simulink model "model"  (Simulink 7.3)
settings: Solver=ode45  StartTime=0.0  StopTime=2  RelTol=1e-3
values from neighbouring files (symbols this model uses):
  C_bp = 0.358    [init.m]
  C_bv = 10.71    [init.m]
  C_ep = 0.668    [init.m]
  C_ev = 20    [init.m]
  C_hp = 0.119    [init.m]
  C_hv = 3.57    [init.m]
  C_la = 19.23    [init.m]
  C_mp = 0.525    [init.m]
  C_mv = 15.71    [init.m]
  C_pa = 0.76    [init.m]
  C_pp = 5.8    [init.m]
  C_pv = 25.37    [init.m]
  C_ra = 31.25    [init.m]
  C_sa = 0.28    [init.m]
  C_sp = 2.05    [init.m]
  C_sv = 61.11    [init.m]
  D_E_max_lv = 2    [init.m]
  D_E_max_rv = 2    [init.m]
  D_R_ep = 2    [init.m]
  D_R_mp = 2    [init.m]
  D_R_sp = 2    [init.m]
  D_T_s = 2    [init.m]
  D_T_v = 0.02    [init.m]
  D_u_ev = 5    [init.m]
  D_u_mv = 5    [init.m]
  D_u_sv = 5    [init.m]
  D_v = 6    [init.m]
  E_max_lv_0 = 2.392    [init.m]
  E_max_rv_0 = 1.412    [init.m]
  f_ab_0 = 1    [init.m]
  f_abmax = 47.78    [init.m]
  f_abmin = 0    [init.m]
  f_ac_max = 17.07    [init.m]
  f_ac_min = 0    [init.m]
  f_ac_n = 3.6    [init.m]
  f_es_0 = 16.11    [init.m]
  f_es_inf = 2.1    [init.m]
  f_es_max = 60    [init.m]
  f_es_min = 0    [init.m]
  f_ev_0 = 3.2    [init.m]
  f_ev_inf = 6.3    [init.m]
  fi_sh = 0    [init.m]
  fi_sp = 0    [init.m]
  fi_v = -0.68    [init.m]
  G_ap = 23.29    [init.m]
  G_E_max_lv = 0.475    [init.m]
  G_E_max_rv = 0.282    [init.m]
  G_R_ep = 1.94    [init.m]
  G_R_mp = 2.47    [init.m]
  G_R_sp = 0.695    [init.m]
  G_T_s = -0.13    [init.m]
  G_T_v = 0.09    [init.m]
  G_u_ev = -74.21    [init.m]
  G_u_mv = -58.29    [init.m]
  G_u_sv = -265.4    [init.m]
  G_v = 0.125    [init.m]
  k_a_b = 11.76    [init.m]
  k_ac = 29.27    [init.m]
  k_e_lv = 0.014    [init.m]
  k_e_rv = 0.011    [init.m]
  k_es = 0.0675    [init.m]
  k_ev = 7.06    [init.m]
  k_r_lv = 0.000375    [init.m]
  k_r_rv = 0.0014    [init.m]
  k_sys = 0.075    [init.m]
  L_pa = 0.00018    [init.m]
  p_as_o2 = 30    [init.m]
  p_as_o2_n = 45    [init.m]
  p_n = 92    [init.m]
  P_o_lv = 1.5    [init.m]
  P_o_rv = 1.5    [init.m]
  R_bp = 6.57    [init.m]
  R_bv = 0.075    [init.m]
  R_ep_0 = 1.655    [init.m]
  R_ev = 0.04    [init.m]
  R_hp = 19.71    [init.m]
  R_hv = 0.224    [init.m]
  R_la = 0.0025    [init.m]
  R_mp_0 = 2.106    [init.m]
  R_mv = 0.05    [init.m]
  R_pa = 0.023    [init.m]
  R_pp = 0.0894    [init.m]
  R_pv = 0.0056    [init.m]
  R_ra = 0.0025    [init.m]
  R_sa = 0.06    [init.m]
  R_sp_0 = 2.49    [init.m]
  R_sv = 0.038    [init.m]
  T_0 = 0.58    [init.m]
  T_sys_0 = 0.5    [init.m]
  tau_c = 2    [init.m]
  tau_E_max_rv = 8    [init.m]
  tau_p = 2    [init.m]
  tau_pb = 2.076    [init.m]
  tau_R_ep = 6    [init.m]
  tau_R_mp = 6    [init.m]
  tau_R_sp = 6    [init.m]
  tau_T_s = 2    [init.m]
  tau_T_v = 1.5    [init.m]
  tau_u_ev = 20    [init.m]
  tau_u_mv = 20    [init.m]
  tau_u_sv = 20    [init.m]
  tau_v = 3    [init.m]
  tau_zb = 6.37    [init.m]
  V_tn = 0.583    [init.m]
  V_tot = 5300    [init.m]
  V_u_bp = 72.13    [init.m]
  V_u_bv = 294.64    [init.m]
  V_u_ep = 134.64    [init.m]
  V_u_ev_0 = 640.73    [init.m]
  V_u_hp = 24    [init.m]
  V_u_hv = 98.21    [init.m]
  V_u_la = 25    [init.m]
  V_u_lv = 16.77    [init.m]
  V_u_mp = 105.8    [init.m]
  V_u_mv_0 = 503.26    [init.m]
  V_u_pa = 0    [init.m]
  V_u_pp = 123    [init.m]
  V_u_pv = 120    [init.m]
  V_u_ra = 25    [init.m]
  V_u_rv = 40.8    [init.m]
  ... (+11 more)
(part 1 of 2)
settings Model: Creator=Mirek Muzny  LastModifiedBy=Mirek Muzny

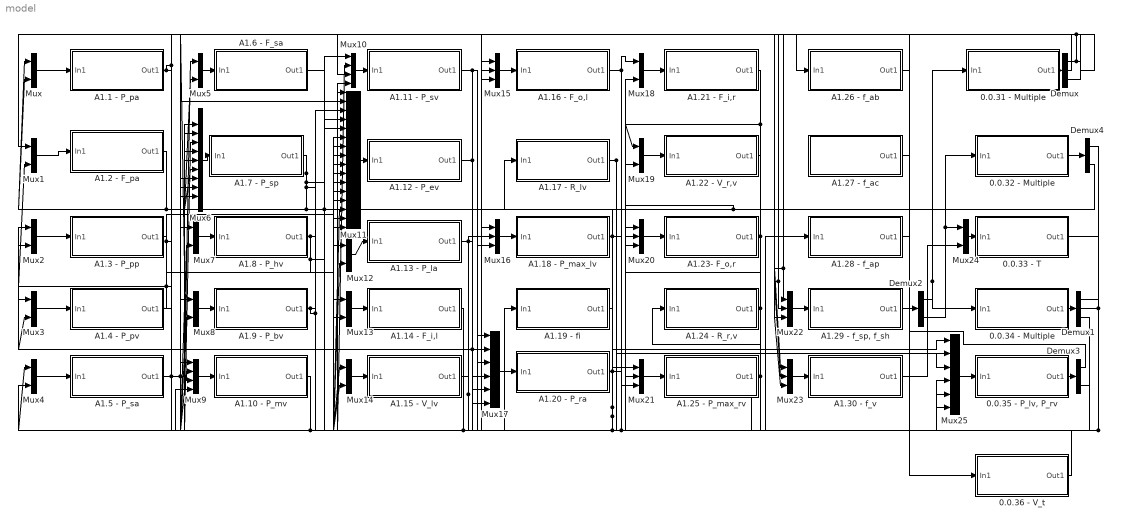
== system model ==
  0.0.31 - Multiple : Subsystem
  0.0.32 - Multiple : Subsystem
  0.0.33 - T : Subsystem
  0.0.34 - Multiple : Subsystem
  "0.0.35 - P_lv, P_rv" : Subsystem
  0.0.36 - V_t : Subsystem
  A1.1 - P_pa : Subsystem
  A1.10 - P_mv : Subsystem
  A1.11 - P_sv : Subsystem
  A1.12 - P_ev : Subsystem
  A1.13 - P_la : Subsystem
  A1.14 - F_i,l : Subsystem
  A1.15 - V_lv : Subsystem
  A1.16 - F_o,l : Subsystem
  A1.17 - R_lv : Subsystem
  A1.18 - P_max_lv : Subsystem
  A1.19 - fi : Subsystem
  A1.2 - F_pa : Subsystem
  A1.20 - P_ra : Subsystem
  A1.21 - F_i,r : Subsystem
  A1.22 - V_r,v : Subsystem
  A1.23- F_o,r : Subsystem
  A1.24 - R_r,v : Subsystem
  A1.25 - P_max_rv : Subsystem
  A1.26 - f_ab : Subsystem
  A1.27 - f_ac : Subsystem
  A1.28 - f_ap : Subsystem
  "A1.29 - f_sp, f_sh" : Subsystem
  A1.3 - P_pp : Subsystem
  "A1.30 - f_v " : Subsystem
  A1.4 - P_pv : Subsystem
  A1.5 - P_sa : Subsystem
  A1.6 - F_sa : Subsystem
  A1.7 - P_sp : Subsystem
  A1.8 - P_hv : Subsystem
  A1.9 - P_bv : Subsystem
  Demux : Demux  Outputs=3
  Demux1 : Demux  Outputs=3
  Demux2 : Demux  Outputs=2
  Demux3 : Demux  Outputs=2
  Demux4 : Demux  Outputs=2
  Mux{,1..5,7..8,12..14,18..19,24} (14 alike) : Mux  Inputs=2
  Mux10 : Mux
  Mux11 : Mux  Inputs=16
  Mux{15..16,20..23} (6 alike) : Mux  Inputs=3
  Mux17 : Mux  Inputs=6
  Mux25 : Mux  Inputs=6
  Mux6 : Mux  Inputs=9
  Mux9 : Mux
  wires:
  Mux/1 -> A1.1 - P_pa/1(In1)
  A1.23- F_o,r/1(Out1) -> Mux/1, Mux19/2, Mux25/6
  A1.2 - F_pa/1(Out1) -> Mux/2, Mux2/2
  Mux1/1 -> A1.2 - F_pa/1(In1)
  A1.1 - P_pa/1(Out1) -> Mux1/1, Mux11/8, Mux20/2
  A1.3 - P_pp/1(Out1) -> Mux1/2, Mux3/1, Mux11/9
  Mux2/1 -> A1.3 - P_pp/1(In1)
  A1.4 - P_pv/1(Out1) -> Mux2/1, Mux11/10, Mux12/1
  Mux3/1 -> A1.4 - P_pv/1(In1)
  A1.13 - P_la/1(Out1) -> Mux3/2, Mux11/11, Mux13/1
  Mux4/1 -> A1.5 - P_sa/1(In1)
  A1.6 - F_sa/1(Out1) -> Mux4/2, Mux6/6
  A1.16 - F_o,l/1(Out1) -> Mux4/1, Mux14/2, Mux25/3
  Mux5/1 -> A1.6 - F_sa/1(In1)
  A1.7 - P_sp/1(Out1) -> Mux5/2, Mux7/1, Mux8/1, Mux9/1, Mux10/1, Mux11/1
  A1.5 - P_sa/1(Out1) -> Mux5/1, Mux11/2, Mux15/2, A1.26 - f_ab/1(In1)
  Mux6/1 -> A1.7 - P_sp/1(In1)
  A1.8 - P_hv/1(Out1) -> Mux6/1, Mux11/4, Mux17/1
  A1.9 - P_bv/1(Out1) -> Mux6/2, Mux11/3, Mux17/2
  A1.10 - P_mv/1(Out1) -> Mux6/3, Mux11/5, Mux17/3
  A1.11 - P_sv/1(Out1) -> Mux6/4, Mux11/6, Mux17/4
  A1.12 - P_ev/1(Out1) -> Mux6/5, Mux17/5
  0.0.31 - Multiple/1(Out1) -> Demux/1
  Demux/2 -> Mux6/7
  Demux/1 -> Mux6/8, Mux9/3, Mux10/3
  Demux/3 -> Mux6/9
  Mux7/1 -> A1.8 - P_hv/1(In1)
  A1.20 - P_ra/1(Out1) -> Mux7/2, Mux8/2, Mux9/2, Mux10/2, Mux11/7, Mux18/1
  Mux8/1 -> A1.9 - P_bv/1(In1)
  Mux9/1 -> A1.10 - P_mv/1(In1)
  0.0.34 - Multiple/1(Out1) -> Demux1/1
  Demux1/1 -> Mux9/4, Mux11/14
  Mux10/1 -> A1.11 - P_sv/1(In1)
  Demux1/2 -> Mux10/4, Mux11/15
  Mux11/1 -> A1.12 - P_ev/1(In1)
  A1.22 - V_r,v/1(Out1) -> Mux11/12, Mux21/2
  A1.15 - V_lv/1(Out1) -> Mux16/2, Mux11/13
  Demux1/3 -> Mux11/16
  Mux12/1 -> A1.13 - P_la/1(In1)
  A1.14 - F_i,l/1(Out1) -> Mux12/2, Mux14/1
  Mux13/1 -> A1.14 - F_i,l/1(In1)
  Mux14/1 -> A1.15 - V_lv/1(In1)
  Mux15/1 -> A1.16 - F_o,l/1(In1)
  A1.18 - P_max_lv/1(Out1) -> Mux15/1, A1.17 - R_lv/1(In1), Mux25/1
  A1.17 - R_lv/1(Out1) -> Mux15/3, Mux25/2
  Mux16/1 -> A1.18 - P_max_lv/1(In1)
  A1.19 - fi/1(Out1) -> Mux16/1, Mux21/1
  0.0.33 - T/1(Out1) -> A1.19 - fi/1(In1)
  Mux17/1 -> A1.20 - P_ra/1(In1)
  A1.21 - F_i,r/1(Out1) -> Mux17/6, Mux19/1
  Mux18/1 -> A1.21 - F_i,r/1(In1)
  Mux19/1 -> A1.22 - V_r,v/1(In1)
  Mux20/1 -> A1.23- F_o,r/1(In1)
  A1.24 - R_r,v/1(Out1) -> Mux20/3, Mux25/5
  A1.25 - P_max_rv/1(Out1) -> A1.24 - R_r,v/1(In1), Mux25/4, Mux20/1
  Mux21/1 -> A1.25 - P_max_rv/1(In1)
  0.0.36 - V_t/1(Out1) -> A1.28 - f_ap/1(In1)
  Mux22/1 -> "A1.29 - f_sp, f_sh"/1(In1)
  A1.26 - f_ab/1(Out1) -> Mux22/1, Mux23/1
  A1.27 - f_ac/1(Out1) -> Mux22/2, Mux23/2, 0.0.36 - V_t/1(In1)
  A1.28 - f_ap/1(Out1) -> Mux22/3, Mux23/3
  Mux23/1 -> "A1.30 - f_v "/1(In1)
  "A1.29 - f_sp, f_sh"/1(Out1) -> Demux2/1
  Demux2/2 -> 0.0.32 - Multiple/1(In1), Mux24/1
  Demux2/1 -> 0.0.31 - Multiple/1(In1), 0.0.34 - Multiple/1(In1)
  Mux24/1 -> 0.0.33 - T/1(In1)
  "A1.30 - f_v "/1(Out1) -> Mux24/2
  "0.0.35 - P_lv, P_rv"/1(Out1) -> Demux3/1
  Mux25/1 -> "0.0.35 - P_lv, P_rv"/1(In1)
  Demux3/2 -> Mux18/2
  Demux3/1 -> Mux13/2
  0.0.32 - Multiple/1(Out1) -> Demux4/1
  Demux4/1 -> Mux21/3
  Demux4/2 -> Mux16/3

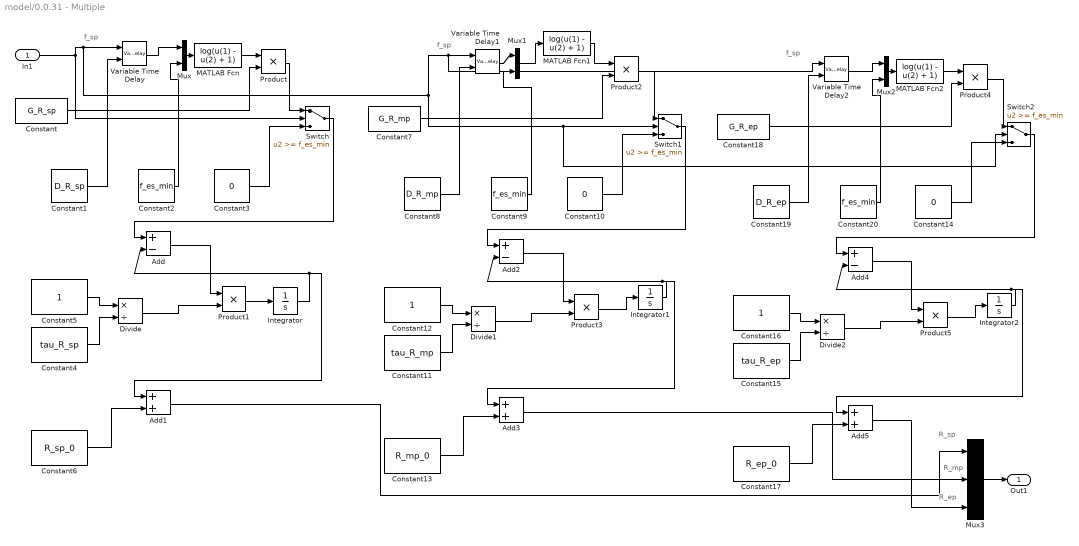
== system model/0.0.31 - Multiple ==
  note: f_sp
  note: f_sp
  note: f_sp
  note: R_sp
  note: R_mp
  note: R_ep
  In1 : Inport  OutDataType=fixdt(1, 16)  OutScaling=2^0
  Add : Sum  Inputs=+-  OutDataType=fixdt(1, 16)  OutScaling=2^-10
  Add1 : Sum  OutDataType=fixdt(1, 16)  OutScaling=2^-10
  Add2 : Sum  Inputs=+-  OutDataType=fixdt(1, 16)  OutScaling=2^-10
  Add3 : Sum  OutDataType=fixdt(1, 16)  OutScaling=2^-10
  Add4 : Sum  Inputs=+-  OutDataType=fixdt(1, 16)  OutScaling=2^-10
  Add5 : Sum  OutDataType=fixdt(1, 16)  OutScaling=2^-10
  Constant : Constant  Value=G_R_sp  OutDataType=fixdt(1, 16)  OutScaling=2^0
  Constant1 : Constant  Value=D_R_sp  OutDataType=fixdt(1, 16)  OutScaling=2^0
  Constant10 : Constant  Value=0  OutDataType=fixdt(1, 16)  OutScaling=2^0
  Constant11 : Constant  Value=tau_R_mp  OutDataType=fixdt(1, 16)  OutScaling=2^0
  Constant12 : Constant  OutDataType=fixdt(1, 16)  OutScaling=2^0
  Constant13 : Constant  Value=R_mp_0  OutDataType=fixdt(1, 16)  OutScaling=2^0
  Constant14 : Constant  Value=0  OutDataType=fixdt(1, 16)  OutScaling=2^0
  Constant15 : Constant  Value=tau_R_ep  OutDataType=fixdt(1, 16)  OutScaling=2^0
  Constant16 : Constant  OutDataType=fixdt(1, 16)  OutScaling=2^0
  Constant17 : Constant  Value=R_ep_0  OutDataType=fixdt(1, 16)  OutScaling=2^0
  Constant18 : Constant  Value=G_R_ep  OutDataType=fixdt(1, 16)  OutScaling=2^0
  Constant19 : Constant  Value=D_R_ep  OutDataType=fixdt(1, 16)  OutScaling=2^0
  Constant2 : Constant  Value=f_es_min  OutDataType=fixdt(1, 16)  OutScaling=2^0
  Constant20 : Constant  Value=f_es_min  OutDataType=fixdt(1, 16)  OutScaling=2^0
  Constant3 : Constant  Value=0  OutDataType=fixdt(1, 16)  OutScaling=2^0
  Constant4 : Constant  Value=tau_R_sp  OutDataType=fixdt(1, 16)  OutScaling=2^0
  Constant5 : Constant  OutDataType=fixdt(1, 16)  OutScaling=2^0
  Constant6 : Constant  Value=R_sp_0  OutDataType=fixdt(1, 16)  OutScaling=2^0
  Constant7 : Constant  Value=G_R_mp  OutDataType=fixdt(1, 16)  OutScaling=2^0
  Constant8 : Constant  Value=D_R_mp  OutDataType=fixdt(1, 16)  OutScaling=2^0
  Constant9 : Constant  Value=f_es_min  OutDataType=fixdt(1, 16)  OutScaling=2^0
  Divide : Product  Inputs=*/  OutDataType=fixdt(1, 16)  OutScaling=2^-10
  Divide1 : Product  Inputs=*/  OutDataType=fixdt(1, 16)  OutScaling=2^-10
  Divide2 : Product  Inputs=*/  OutDataType=fixdt(1, 16)  OutScaling=2^-10
  Integrator : Integrator  InitialCondition=100
  Integrator1 : Integrator  InitialCondition=1
  Integrator2 : Integrator  InitialCondition=1
  MATLAB Fcn : MATLABFcn  MATLABFcn=log(u(1) - u(2) + 1)
  MATLAB Fcn1 : MATLABFcn  MATLABFcn=log(u(1) - u(2) + 1)
  MATLAB Fcn2 : MATLABFcn  MATLABFcn=log(u(1) - u(2) + 1)
  Mux : Mux  Inputs=2
  Mux1 : Mux  Inputs=2
  Mux2 : Mux  Inputs=2
  Mux3 : Mux  Inputs=3
  Product{,2..5} (5 alike) : Product  OutDataType=fixdt(1, 16)  OutScaling=2^0  RndMeth=Zero
  Product1 : Product  OutMin=[1]  OutDataType=fixdt(1, 16)  OutScaling=2^0  RndMeth=Zero
  Switch : Switch  Threshold=f_es_min  OutDataType=fixdt(1, 16)  OutScaling=2^0
  Switch1 : Switch  Threshold=f_es_min  OutDataType=fixdt(1, 16)  OutScaling=2^0
  Switch2 : Switch  Threshold=f_es_min  OutDataType=fixdt(1, 16)  OutScaling=2^0
  Variable Time Delay : VariableTransportDelay  MaximumDelay=10
  Variable Time Delay1 : VariableTransportDelay  MaximumDelay=10
  Variable Time Delay2 : VariableTransportDelay  MaximumDelay=10
  Out1 : Outport  OutDataType=fixdt(1, 16)  OutScaling=2^0
  wires:
  Constant/1 -> Product/2
  Constant1/1 -> Variable Time Delay/2
  Mux/1 -> MATLAB Fcn/1
  Variable Time Delay/1 -> Mux/1
  Constant2/1 -> Mux/2
  MATLAB Fcn/1 -> Product/1
  Product/1 -> Switch/1
  Constant3/1 -> Switch/3
  Switch/1 -> Add/1
  Integrator/1 -> Add/2, Add1/1
  Add/1 -> Product1/1
  Constant4/1 -> Divide/2
  Constant5/1 -> Divide/1
  Divide/1 -> Product1/2
  Product1/1 -> Integrator/1
  In1/1 -> Switch/2, Variable Time Delay/1, Variable Time Delay1/1, Variable Time Delay2/1, Switch1/2, Switch2/2
  Constant6/1 -> Add1/2
  Constant7/1 -> Product2/2
  Constant8/1 -> Variable Time Delay1/2
  Mux1/1 -> MATLAB Fcn1/1
  Variable Time Delay1/1 -> Mux1/1
  Constant9/1 -> Mux1/2
  MATLAB Fcn1/1 -> Product2/1
  Product2/1 -> Switch1/1
  Constant10/1 -> Switch1/3
  Switch1/1 -> Add2/1
  Integrator1/1 -> Add2/2, Add3/1
  Add2/1 -> Product3/1
  Constant11/1 -> Divide1/2
  Constant12/1 -> Divide1/1
  Divide1/1 -> Product3/2
  Product3/1 -> Integrator1/1
  Constant13/1 -> Add3/2
  Constant18/1 -> Product4/2
  Constant19/1 -> Variable Time Delay2/2
  Mux2/1 -> MATLAB Fcn2/1
  Variable Time Delay2/1 -> Mux2/1
  Constant20/1 -> Mux2/2
  MATLAB Fcn2/1 -> Product4/1
  Product4/1 -> Switch2/1
  Constant14/1 -> Switch2/3
  Switch2/1 -> Add4/1
  Integrator2/1 -> Add4/2, Add5/1
  Add4/1 -> Product5/1
  Constant15/1 -> Divide2/2
  Constant16/1 -> Divide2/1
  Divide2/1 -> Product5/2
  Product5/1 -> Integrator2/1
  Constant17/1 -> Add5/2
  Add1/1 -> Mux3/1
  Add3/1 -> Mux3/2
  Add5/1 -> Mux3/3
  Mux3/1 -> Out1/1

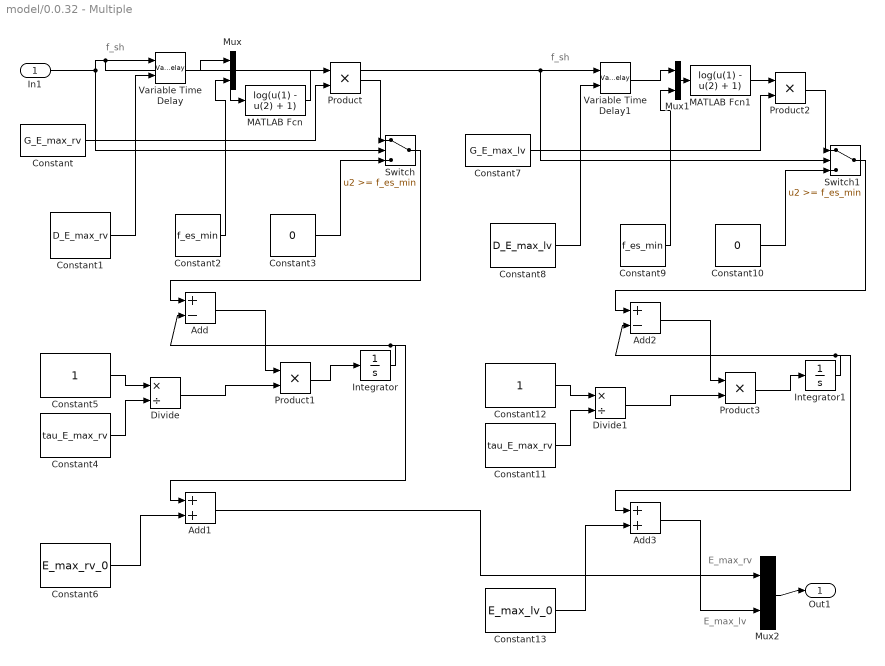
== system model/0.0.32 - Multiple ==
  note: f_sh
  note: f_sh
  note: E_max_rv
  note: E_max_lv
  In1 : Inport  OutDataType=fixdt(1, 16)  OutScaling=2^0
  Add : Sum  Inputs=+-  OutDataType=fixdt(1, 16)  OutScaling=2^-10
  Add1 : Sum  OutDataType=fixdt(1, 16)  OutScaling=2^-10
  Add2 : Sum  Inputs=+-  OutDataType=fixdt(1, 16)  OutScaling=2^-10
  Add3 : Sum  OutDataType=fixdt(1, 16)  OutScaling=2^-10
  Constant : Constant  Value=G_E_max_rv  OutDataType=fixdt(1, 16)  OutScaling=2^0
  Constant1 : Constant  Value=D_E_max_rv  OutDataType=fixdt(1, 16)  OutScaling=2^0
  Constant10 : Constant  Value=0  OutDataType=fixdt(1, 16)  OutScaling=2^0
  Constant11 : Constant  Value=tau_E_max_rv  OutDataType=fixdt(1, 16)  OutScaling=2^0
  Constant12 : Constant  OutDataType=fixdt(1, 16)  OutScaling=2^0
  Constant13 : Constant  Value=E_max_lv_0  OutDataType=fixdt(1, 16)  OutScaling=2^0
  Constant2 : Constant  Value=f_es_min  OutDataType=fixdt(1, 16)  OutScaling=2^0
  Constant3 : Constant  Value=0  OutDataType=fixdt(1, 16)  OutScaling=2^0
  Constant4 : Constant  Value=tau_E_max_rv  OutDataType=fixdt(1, 16)  OutScaling=2^0
  Constant5 : Constant  OutDataType=fixdt(1, 16)  OutScaling=2^0
  Constant6 : Constant  Value=E_max_rv_0  OutDataType=fixdt(1, 16)  OutScaling=2^0
  Constant7 : Constant  Value=G_E_max_lv  OutDataType=fixdt(1, 16)  OutScaling=2^0
  Constant8 : Constant  Value=D_E_max_lv  OutDataType=fixdt(1, 16)  OutScaling=2^0
  Constant9 : Constant  Value=f_es_min  OutDataType=fixdt(1, 16)  OutScaling=2^0
  Divide : Product  Inputs=*/  OutDataType=fixdt(1, 16)  OutScaling=2^-10
  Divide1 : Product  Inputs=*/  OutDataType=fixdt(1, 16)  OutScaling=2^-10
  Integrator : Integrator  InitialCondition=1
  Integrator1 : Integrator  InitialCondition=1
  MATLAB Fcn : MATLABFcn  MATLABFcn=log(u(1) - u(2) + 1)
  MATLAB Fcn1 : MATLABFcn  MATLABFcn=log(u(1) - u(2) + 1)
  Mux : Mux  Inputs=2
  Mux1 : Mux  Inputs=2
  Mux2 : Mux  Inputs=2
  Product{,1..3} (4 alike) : Product  OutDataType=fixdt(1, 16)  OutScaling=2^0  RndMeth=Zero
  Switch : Switch  Threshold=f_es_min  OutDataType=fixdt(1, 16)  OutScaling=2^0
  Switch1 : Switch  Threshold=f_es_min  OutDataType=fixdt(1, 16)  OutScaling=2^0
  Variable Time Delay : VariableTransportDelay  MaximumDelay=10
  Variable Time Delay1 : VariableTransportDelay  MaximumDelay=10
  Out1 : Outport  OutDataType=fixdt(1, 16)  OutScaling=2^0
  wires:
  Constant/1 -> Product/2
  Constant1/1 -> Variable Time Delay/2
  Mux/1 -> MATLAB Fcn/1
  Variable Time Delay/1 -> Mux/1
  Constant2/1 -> Mux/2
  MATLAB Fcn/1 -> Product/1
  Product/1 -> Switch/1
  Constant3/1 -> Switch/3
  Switch/1 -> Add/1
  Integrator/1 -> Add/2, Add1/1
  Add/1 -> Product1/1
  Constant4/1 -> Divide/2
  Constant5/1 -> Divide/1
  Divide/1 -> Product1/2
  Product1/1 -> Integrator/1
  In1/1 -> Switch/2, Variable Time Delay/1, Switch1/2, Variable Time Delay1/1
  Constant6/1 -> Add1/2
  Constant7/1 -> Product2/2
  Constant8/1 -> Variable Time Delay1/2
  Mux1/1 -> MATLAB Fcn1/1
  Variable Time Delay1/1 -> Mux1/1
  Constant9/1 -> Mux1/2
  MATLAB Fcn1/1 -> Product2/1
  Product2/1 -> Switch1/1
  Constant10/1 -> Switch1/3
  Switch1/1 -> Add2/1
  Integrator1/1 -> Add2/2, Add3/1
  Add2/1 -> Product3/1
  Constant11/1 -> Divide1/2
  Constant12/1 -> Divide1/1
  Divide1/1 -> Product3/2
  Product3/1 -> Integrator1/1
  Constant13/1 -> Add3/2
  Add1/1 -> Mux2/1
  Add3/1 -> Mux2/2
  Mux2/1 -> Out1/1

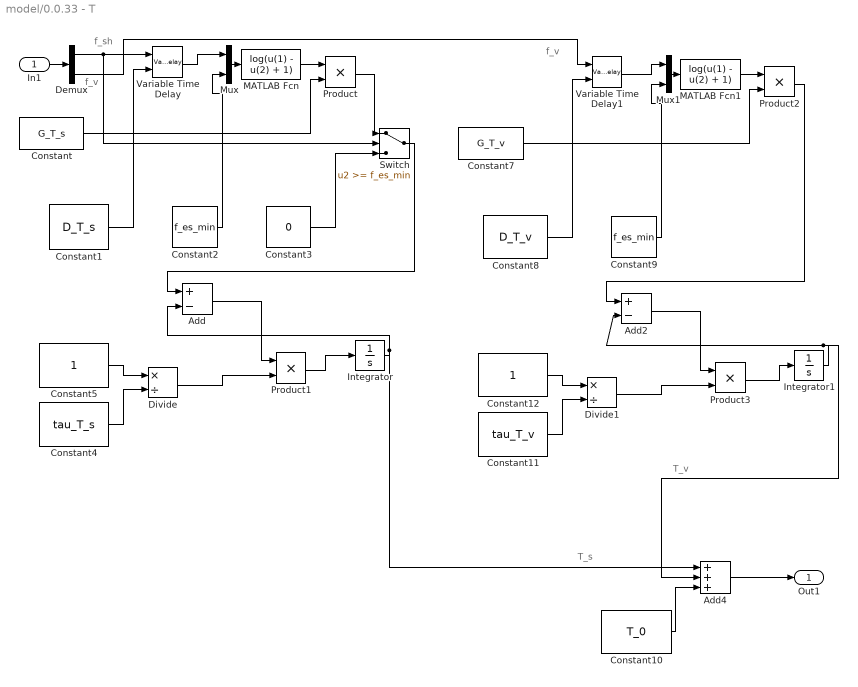
== system model/0.0.33 - T ==
  note: f_sh
  note: f_v
  note: f_v
  note: T_s
  note: T_v
  In1 : Inport  OutDataType=fixdt(1, 16)  OutScaling=2^0
  Add : Sum  Inputs=+-  OutDataType=fixdt(1, 16)  OutScaling=2^-10
  Add2 : Sum  Inputs=+-  OutDataType=fixdt(1, 16)  OutScaling=2^-10
  Add4 : Sum  Inputs=+++  OutDataType=fixdt(1, 16)  OutScaling=2^-10
  Constant : Constant  Value=G_T_s  OutDataType=fixdt(1, 16)  OutScaling=2^0
  Constant1 : Constant  Value=D_T_s  OutDataType=fixdt(1, 16)  OutScaling=2^0
  Constant10 : Constant  Value=T_0  OutDataType=fixdt(1, 16)  OutScaling=2^0
  Constant11 : Constant  Value=tau_T_v  OutDataType=fixdt(1, 16)  OutScaling=2^0
  Constant12 : Constant  OutDataType=fixdt(1, 16)  OutScaling=2^0
  Constant2 : Constant  Value=f_es_min  OutDataType=fixdt(1, 16)  OutScaling=2^0
  Constant3 : Constant  Value=0  OutDataType=fixdt(1, 16)  OutScaling=2^0
  Constant4 : Constant  Value=tau_T_s  OutDataType=fixdt(1, 16)  OutScaling=2^0
  Constant5 : Constant  OutDataType=fixdt(1, 16)  OutScaling=2^0
  Constant7 : Constant  Value=G_T_v  OutDataType=fixdt(1, 16)  OutScaling=2^0
  Constant8 : Constant  Value=D_T_v  OutDataType=fixdt(1, 16)  OutScaling=2^0
  Constant9 : Constant  Value=f_es_min  OutDataType=fixdt(1, 16)  OutScaling=2^0
  Demux : Demux  Outputs=2
  Divide : Product  Inputs=*/  OutDataType=fixdt(1, 16)  OutScaling=2^-10
  Divide1 : Product  Inputs=*/  OutDataType=fixdt(1, 16)  OutScaling=2^-10
  Integrator : Integrator  InitialCondition=1
  Integrator1 : Integrator  InitialCondition=1
  MATLAB Fcn : MATLABFcn  MATLABFcn=log(u(1) - u(2) + 1)
  MATLAB Fcn1 : MATLABFcn  MATLABFcn=log(u(1) - u(2) + 1)
  Mux : Mux  Inputs=2
  Mux1 : Mux  Inputs=2
  Product{,1..3} (4 alike) : Product  OutDataType=fixdt(1, 16)  OutScaling=2^0  RndMeth=Zero
  Switch : Switch  Threshold=f_es_min  OutDataType=fixdt(1, 16)  OutScaling=2^0
  Variable Time Delay : VariableTransportDelay  MaximumDelay=10
  Variable Time Delay1 : VariableTransportDelay  MaximumDelay=10
  Out1 : Outport  OutDataType=fixdt(1, 16)  OutScaling=2^0
  wires:
  Constant/1 -> Product/2
  Constant1/1 -> Variable Time Delay/2
  Mux/1 -> MATLAB Fcn/1
  Variable Time Delay/1 -> Mux/1
  Constant2/1 -> Mux/2
  MATLAB Fcn/1 -> Product/1
  Product/1 -> Switch/1
  Constant3/1 -> Switch/3
  Switch/1 -> Add/1
  Integrator/1 -> Add/2, Add4/1
  Add/1 -> Product1/1
  Constant4/1 -> Divide/2
  Constant5/1 -> Divide/1
  Divide/1 -> Product1/2
  Product1/1 -> Integrator/1
  Constant7/1 -> Product2/2
  Constant8/1 -> Variable Time Delay1/2
  Mux1/1 -> MATLAB Fcn1/1
  Variable Time Delay1/1 -> Mux1/1
  Constant9/1 -> Mux1/2
  MATLAB Fcn1/1 -> Product2/1
  Integrator1/1 -> Add2/2, Add4/2
  Add2/1 -> Product3/1
  Constant11/1 -> Divide1/2
  Constant12/1 -> Divide1/1
  Divide1/1 -> Product3/2
  Product3/1 -> Integrator1/1
  In1/1 -> Demux/1
  Product2/1 -> Add2/1
  Demux/2 -> Variable Time Delay1/1
  Demux/1 -> Variable Time Delay/1, Switch/2
  Constant10/1 -> Add4/3
  Add4/1 -> Out1/1

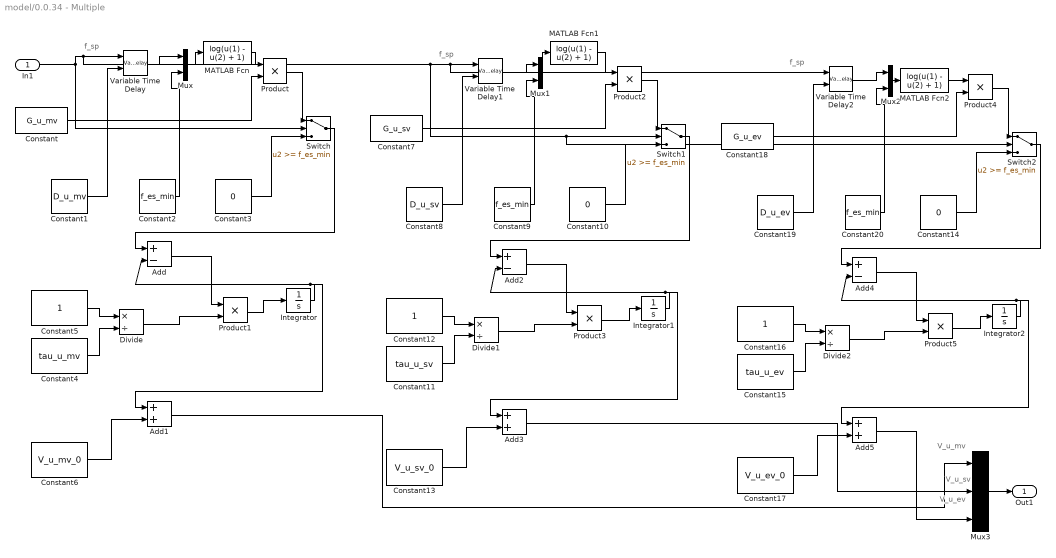
== system model/0.0.34 - Multiple ==
  note: f_sp
  note: f_sp
  note: f_sp
  note: V_u_mv
  note: V_u_sv
  note: V_u_ev
  In1 : Inport  OutDataType=fixdt(1, 16)  OutScaling=2^0
  Add : Sum  Inputs=+-  OutDataType=fixdt(1, 16)  OutScaling=2^-10
  Add1 : Sum  OutDataType=fixdt(1, 16)  OutScaling=2^-10
  Add2 : Sum  Inputs=+-  OutDataType=fixdt(1, 16)  OutScaling=2^-10
  Add3 : Sum  OutDataType=fixdt(1, 16)  OutScaling=2^-10
  Add4 : Sum  Inputs=+-  OutDataType=fixdt(1, 16)  OutScaling=2^-10
  Add5 : Sum  OutDataType=fixdt(1, 16)  OutScaling=2^-10
  Constant : Constant  Value=G_u_mv  OutDataType=fixdt(1, 16)  OutScaling=2^0
  Constant1 : Constant  Value=D_u_mv  OutDataType=fixdt(1, 16)  OutScaling=2^0
  Constant10 : Constant  Value=0  OutDataType=fixdt(1, 16)  OutScaling=2^0
  Constant11 : Constant  Value=tau_u_sv  OutDataType=fixdt(1, 16)  OutScaling=2^0
  Constant12 : Constant  OutDataType=fixdt(1, 16)  OutScaling=2^0
  Constant13 : Constant  Value=V_u_sv_0  OutDataType=fixdt(1, 16)  OutScaling=2^0
  Constant14 : Constant  Value=0  OutDataType=fixdt(1, 16)  OutScaling=2^0
  Constant15 : Constant  Value=tau_u_ev  OutDataType=fixdt(1, 16)  OutScaling=2^0
  Constant16 : Constant  OutDataType=fixdt(1, 16)  OutScaling=2^0
  Constant17 : Constant  Value=V_u_ev_0  OutDataType=fixdt(1, 16)  OutScaling=2^0
  Constant18 : Constant  Value=G_u_ev  OutDataType=fixdt(1, 16)  OutScaling=2^0
  Constant19 : Constant  Value=D_u_ev  OutDataType=fixdt(1, 16)  OutScaling=2^0
  Constant2 : Constant  Value=f_es_min  OutDataType=fixdt(1, 16)  OutScaling=2^0
  Constant20 : Constant  Value=f_es_min  OutDataType=fixdt(1, 16)  OutScaling=2^0
  Constant3 : Constant  Value=0  OutDataType=fixdt(1, 16)  OutScaling=2^0
  Constant4 : Constant  Value=tau_u_mv  OutDataType=fixdt(1, 16)  OutScaling=2^0
  Constant5 : Constant  OutDataType=fixdt(1, 16)  OutScaling=2^0
  Constant6 : Constant  Value=V_u_mv_0  OutDataType=fixdt(1, 16)  OutScaling=2^0
  Constant7 : Constant  Value=G_u_sv  OutDataType=fixdt(1, 16)  OutScaling=2^0
  Constant8 : Constant  Value=D_u_sv  OutDataType=fixdt(1, 16)  OutScaling=2^0
  Constant9 : Constant  Value=f_es_min  OutDataType=fixdt(1, 16)  OutScaling=2^0
  Divide : Product  Inputs=*/  OutDataType=fixdt(1, 16)  OutScaling=2^-10
  Divide1 : Product  Inputs=*/  OutDataType=fixdt(1, 16)  OutScaling=2^-10
  Divide2 : Product  Inputs=*/  OutDataType=fixdt(1, 16)  OutScaling=2^-10
  Integrator : Integrator  InitialCondition=1
  Integrator1 : Integrator  InitialCondition=1
  Integrator2 : Integrator  InitialCondition=1
  MATLAB Fcn : MATLABFcn  MATLABFcn=log(u(1) - u(2) + 1)
  MATLAB Fcn1 : MATLABFcn  MATLABFcn=log(u(1) - u(2) + 1)
  MATLAB Fcn2 : MATLABFcn  MATLABFcn=log(u(1) - u(2) + 1)
  Mux : Mux  Inputs=2
  Mux1 : Mux  Inputs=2
  Mux2 : Mux  Inputs=2
  Mux3 : Mux  Inputs=3
  Product{,1..5} (6 alike) : Product  OutDataType=fixdt(1, 16)  OutScaling=2^0  RndMeth=Zero
  Switch : Switch  Threshold=f_es_min  OutDataType=fixdt(1, 16)  OutScaling=2^0
  Switch1 : Switch  Threshold=f_es_min  OutDataType=fixdt(1, 16)  OutScaling=2^0
  Switch2 : Switch  Threshold=f_es_min  OutDataType=fixdt(1, 16)  OutScaling=2^0
  Variable Time Delay : VariableTransportDelay  MaximumDelay=10
  Variable Time Delay1 : VariableTransportDelay  MaximumDelay=10
  Variable Time Delay2 : VariableTransportDelay  MaximumDelay=10
  Out1 : Outport  OutDataType=fixdt(1, 16)  OutScaling=2^0
  wires:
  Constant/1 -> Product/2
  Constant1/1 -> Variable Time Delay/2
  Mux/1 -> MATLAB Fcn/1
  Variable Time Delay/1 -> Mux/1
  Constant2/1 -> Mux/2
  MATLAB Fcn/1 -> Product/1
  Product/1 -> Switch/1
  Constant3/1 -> Switch/3
  Switch/1 -> Add/1
  Integrator/1 -> Add/2, Add1/1
  Add/1 -> Product1/1
  Constant4/1 -> Divide/2
  Constant5/1 -> Divide/1
  Divide/1 -> Product1/2
  Product1/1 -> Integrator/1
  In1/1 -> Switch/2, Variable Time Delay/1, Variable Time Delay1/1, Variable Time Delay2/1, Switch1/2, Switch2/2
  Constant6/1 -> Add1/2
  Constant7/1 -> Product2/2
  Constant8/1 -> Variable Time Delay1/2
  Mux1/1 -> MATLAB Fcn1/1
  Variable Time Delay1/1 -> Mux1/1
  Constant9/1 -> Mux1/2
  MATLAB Fcn1/1 -> Product2/1
  Product2/1 -> Switch1/1
  Constant10/1 -> Switch1/3
  Switch1/1 -> Add2/1
  Integrator1/1 -> Add2/2, Add3/1
  Add2/1 -> Product3/1
  Constant11/1 -> Divide1/2
  Constant12/1 -> Divide1/1
  Divide1/1 -> Product3/2
  Product3/1 -> Integrator1/1
  Constant13/1 -> Add3/2
  Constant18/1 -> Product4/2
  Constant19/1 -> Variable Time Delay2/2
  Mux2/1 -> MATLAB Fcn2/1
  Variable Time Delay2/1 -> Mux2/1
  Constant20/1 -> Mux2/2
  MATLAB Fcn2/1 -> Product4/1
  Product4/1 -> Switch2/1
  Constant14/1 -> Switch2/3
  Switch2/1 -> Add4/1
  Integrator2/1 -> Add4/2, Add5/1
  Add4/1 -> Product5/1
  Constant15/1 -> Divide2/2
  Constant16/1 -> Divide2/1
  Divide2/1 -> Product5/2
  Product5/1 -> Integrator2/1
  Constant17/1 -> Add5/2
  Add1/1 -> Mux3/1
  Add3/1 -> Mux3/2
  Add5/1 -> Mux3/3
  Mux3/1 -> Out1/1

== system model/0.0.35 - P_lv, P_rv ==
  note: P_max_lv
  note: R_lv
  note: F_ol
  note: P_max_rv
  note: R_rv
  note: F_or
  note: P_lv
  note: P_rv
  In1 : Inport  OutDataType=fixdt(1, 16)  OutScaling=2^0
  Add : Sum  Inputs=+-  OutDataType=fixdt(1, 16)  OutScaling=2^-10
  Add1 : Sum  Inputs=+-  OutDataType=fixdt(1, 16)  OutScaling=2^-10
  Demux : Demux  Outputs=6
  Mux : Mux  Inputs=2
  Product : Product  OutDataType=fixdt(1, 16)  OutScaling=2^0  RndMeth=Zero
  Product1 : Product  OutDataType=fixdt(1, 16)  OutScaling=2^0  RndMeth=Zero
  Out1 : Outport  OutDataType=fixdt(1, 16)  OutScaling=2^0
  wires:
  In1/1 -> Demux/1
  Demux/2 -> Product/1
  Demux/3 -> Product/2
  Product/1 -> Add/2
  Demux/1 -> Add/1
  Demux/6 -> Product1/2
  Demux/5 -> Product1/1
  Demux/4 -> Add1/1
  Product1/1 -> Add1/2
  Add/1 -> Mux/1
  Add1/1 -> Mux/2
  Mux/1 -> Out1/1

== system model/0.0.36 - V_t ==
  In1 : Inport  OutDataType=fixdt(1, 16)  OutScaling=2^0
  Add : Sum  OutDataType=fixdt(1, 16)  OutScaling=2^-10
  Add1 : Sum  Inputs=+-  OutDataType=fixdt(1, 16)  OutScaling=2^-10
  Add2 : Sum  Inputs=+-  OutDataType=fixdt(1, 16)  OutScaling=2^-10
  Constant : Constant  Value=V_tn  OutDataType=fixdt(1, 16)  OutScaling=2^0
  Constant1 : Constant  Value=tau_v  OutDataType=fixdt(1, 16)  OutScaling=2^0
  Constant2 : Constant  Value=D_v  OutDataType=fixdt(1, 16)  OutScaling=2^0
  Constant3 : Constant  Value=f_ac_n  OutDataType=fixdt(1, 16)  OutScaling=2^0
  Constant4 : Constant  Value=G_v  OutDataType=fixdt(1, 16)  OutScaling=2^0
  Divide : Product  Inputs=*/  OutDataType=fixdt(1, 16)  OutScaling=2^-10
  Integrator : Integrator  InitialCondition=1
  Product : Product  OutDataType=fixdt(1, 16)  OutScaling=2^0  RndMeth=Zero
  Variable Time Delay : VariableTransportDelay  MaximumDelay=10
  Out1 : Outport  OutDataType=fixdt(1, 16)  OutScaling=2^0
  wires:
  Constant/1 -> Add/1
  Integrator/1 -> Add/2, Add1/2
  Add/1 -> Out1/1
  Constant2/1 -> Variable Time Delay/2
  In1/1 -> Variable Time Delay/1
  Variable Time Delay/1 -> Add2/1
  Constant3/1 -> Add2/2
  Add2/1 -> Product/1
  Constant4/1 -> Product/2
  Product/1 -> Add1/1
  Add1/1 -> Divide/1
  Constant1/1 -> Divide/2
  Divide/1 -> Integrator/1

== system model/A1.1 - P_pa ==
  note: Fo,r
  note: F pa
  In1 : Inport  OutDataType=fixdt(1, 16)  OutScaling=2^0
  Constant : Constant  Value=C_pa  OutDataType=fixdt(1, 16)  OutScaling=2^0
  Demux : Demux  Outputs=2
  Divide : Product  Inputs=*/  OutDataType=fixdt(1, 16)  OutScaling=2^-10
  Integrator : Integrator  InitialCondition=1
  Subtract : Sum  Inputs=+-  OutDataType=fixdt(1, 16)  OutScaling=2^-10
  Out1 : Outport  OutDataType=fixdt(1, 16)  OutScaling=2^0
  wires:
  In1/1 -> Demux/1
  Demux/1 -> Subtract/1
  Demux/2 -> Subtract/2
  Subtract/1 -> Divide/1
  Constant/1 -> Divide/2
  Divide/1 -> Integrator/1
  Integrator/1 -> Out1/1

== system model/A1.10 - P_mv ==
  note: P_sp
  note: P_ra
  note: R_mp
  note: dV_u_mv/dt
  In1 : Inport  OutDataType=fixdt(1, 16)  OutScaling=2^0
  Constant : Constant  Value=R_mv  OutDataType=fixdt(1, 16)  OutScaling=2^0
  Constant1 : Constant  Value=C_mv  OutDataType=fixdt(1, 16)  OutScaling=2^0
  Demux : Demux
  Derivative : Derivative
  Divide : Product  Inputs=*/  OutDataType=fixdt(1, 16)  OutScaling=2^-10
  Divide1 : Product  Inputs=*/  OutDataType=fixdt(1, 16)  OutScaling=2^-10
  Divide2 : Product  Inputs=*/  OutDataType=fixdt(1, 16)  OutScaling=2^-10
  Integrator : Integrator  InitialCondition=1
  Subtract : Sum  Inputs=+-  OutDataType=fixdt(1, 16)  OutScaling=2^-10
  Subtract1 : Sum  Inputs=+-  OutDataType=fixdt(1, 16)  OutScaling=2^-10
  Subtract2 : Sum  Inputs=++-  OutDataType=fixdt(1, 16)  OutScaling=2^-10
  Out1 : Outport  OutDataType=fixdt(1, 16)  OutScaling=2^0
  wires:
  In1/1 -> Demux/1
  Demux/1 -> Subtract/1
  Subtract/1 -> Divide/1
  Subtract1/1 -> Divide1/1
  Constant/1 -> Divide1/2
  Divide/1 -> Subtract2/1
  Divide1/1 -> Subtract2/2
  Subtract2/1 -> Divide2/1
  Constant1/1 -> Divide2/2
  Divide2/1 -> Integrator/1
  Integrator/1 -> Subtract/2, Subtract1/1, Out1/1
  Demux/2 -> Subtract1/2
  Demux/3 -> Divide/2
  Demux/4 -> Derivative/1
  Derivative/1 -> Subtract2/3

== system model/A1.11 - P_sv ==
  note: P_sp
  note: P_ra
  note: R_sp
  note: dV_u_sv/dt
  In1 : Inport  OutDataType=fixdt(1, 16)  OutScaling=2^0
  Constant : Constant  Value=R_sv  OutDataType=fixdt(1, 16)  OutScaling=2^0
  Constant1 : Constant  Value=C_sv  OutDataType=fixdt(1, 16)  OutScaling=2^0
  Demux : Demux
  Derivative : Derivative
  Divide : Product  Inputs=*/  OutDataType=fixdt(1, 16)  OutScaling=2^-10
  Divide1 : Product  Inputs=*/  OutDataType=fixdt(1, 16)  OutScaling=2^-10
  Divide2 : Product  Inputs=*/  OutDataType=fixdt(1, 16)  OutScaling=2^-10
  Integrator : Integrator  InitialCondition=1
  Subtract : Sum  Inputs=+-  OutDataType=fixdt(1, 16)  OutScaling=2^-10
  Subtract1 : Sum  Inputs=+-  OutDataType=fixdt(1, 16)  OutScaling=2^-10
  Subtract2 : Sum  Inputs=++-  OutDataType=fixdt(1, 16)  OutScaling=2^-10
  Out1 : Outport  OutDataType=fixdt(1, 16)  OutScaling=2^0
  wires:
  In1/1 -> Demux/1
  Demux/1 -> Subtract/1
  Subtract/1 -> Divide/1
  Subtract1/1 -> Divide1/1
  Constant/1 -> Divide1/2
  Divide/1 -> Subtract2/1
  Divide1/1 -> Subtract2/2
  Subtract2/1 -> Divide2/1
  Constant1/1 -> Divide2/2
  Divide2/1 -> Integrator/1
  Integrator/1 -> Subtract/2, Subtract1/1, Out1/1
  Demux/2 -> Subtract1/2
  Demux/3 -> Divide/2
  Demux/4 -> Derivative/1
  Derivative/1 -> Subtract2/3

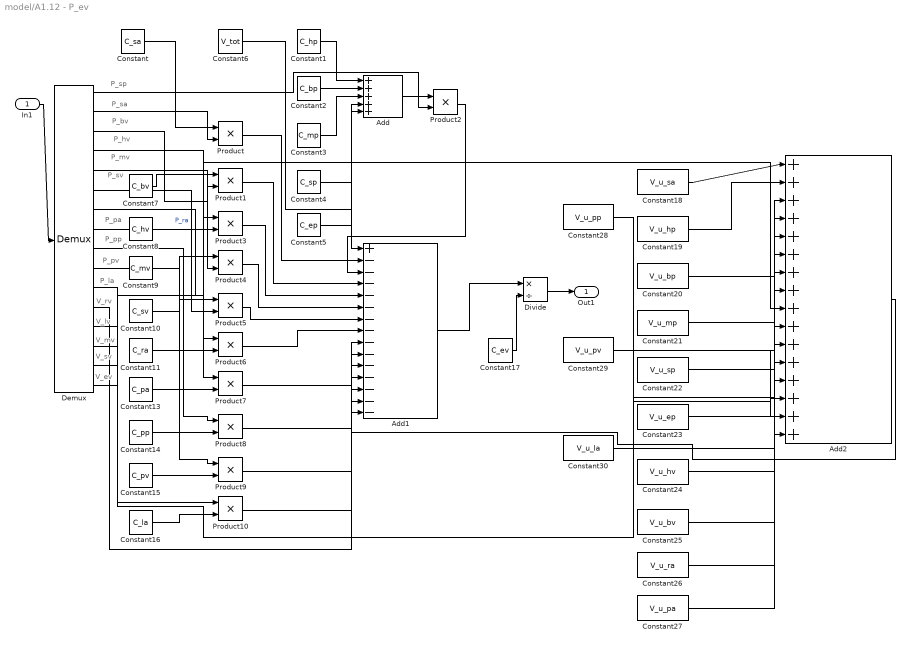
== system model/A1.12 - P_ev ==
  note: P_sp
  note: P_sa
  note: P_bv
  note: P_hv
  note: P_mv
  note: P_sv
  note: P_pa
  note: P_pp
  note: P_pv
  note: P_la
  note: V_rv
  note: V_lv
  note: V_mv
  note: V_sv
  note: V_ev
  In1 : Inport  OutDataType=fixdt(1, 16)  OutScaling=2^0
  Add : Sum  Inputs=+++++  OutDataType=fixdt(1, 16)  OutScaling=2^-10
  Add1 : Sum  Inputs=+--------------  OutDataType=fixdt(1, 16)  OutScaling=2^-10
  Add2 : Sum  Inputs=++++++++++++++++  OutDataType=fixdt(1, 16)  OutScaling=2^-10
  Constant : Constant  Value=C_sa  OutDataType=fixdt(1, 16)  OutScaling=2^0
  Constant1 : Constant  Value=C_hp  OutDataType=fixdt(1, 16)  OutScaling=2^0
  Constant10 : Constant  Value=C_sv  OutDataType=fixdt(1, 16)  OutScaling=2^0
  Constant11 : Constant  Value=C_ra  OutDataType=fixdt(1, 16)  OutScaling=2^0
  Constant13 : Constant  Value=C_pa  OutDataType=fixdt(1, 16)  OutScaling=2^0
  Constant14 : Constant  Value=C_pp  OutDataType=fixdt(1, 16)  OutScaling=2^0
  Constant15 : Constant  Value=C_pv  OutDataType=fixdt(1, 16)  OutScaling=2^0
  Constant16 : Constant  Value=C_la  OutDataType=fixdt(1, 16)  OutScaling=2^0
  Constant17 : Constant  Value=C_ev  OutDataType=fixdt(1, 16)  OutScaling=2^0
  Constant18 : Constant  Value=V_u_sa  OutDataType=fixdt(1, 16)  OutScaling=2^0
  Constant19 : Constant  Value=V_u_hp  OutDataType=fixdt(1, 16)  OutScaling=2^0
  Constant2 : Constant  Value=C_bp  OutDataType=fixdt(1, 16)  OutScaling=2^0
  Constant20 : Constant  Value=V_u_bp  OutDataType=fixdt(1, 16)  OutScaling=2^0
  Constant21 : Constant  Value=V_u_mp  OutDataType=fixdt(1, 16)  OutScaling=2^0
  Constant22 : Constant  Value=V_u_sp  OutDataType=fixdt(1, 16)  OutScaling=2^0
  Constant23 : Constant  Value=V_u_ep  OutDataType=fixdt(1, 16)  OutScaling=2^0
  Constant24 : Constant  Value=V_u_hv  OutDataType=fixdt(1, 16)  OutScaling=2^0
  Constant25 : Constant  Value=V_u_bv  OutDataType=fixdt(1, 16)  OutScaling=2^0
  Constant26 : Constant  Value=V_u_ra  OutDataType=fixdt(1, 16)  OutScaling=2^0
  Constant27 : Constant  Value=V_u_pa  OutDataType=fixdt(1, 16)  OutScaling=2^0
  Constant28 : Constant  Value=V_u_pp  OutDataType=fixdt(1, 16)  OutScaling=2^0
  Constant29 : Constant  Value=V_u_pv  OutDataType=fixdt(1, 16)  OutScaling=2^0
  Constant3 : Constant  Value=C_mp  OutDataType=fixdt(1, 16)  OutScaling=2^0
  Constant30 : Constant  Value=V_u_la  OutDataType=fixdt(1, 16)  OutScaling=2^0
  Constant4 : Constant  Value=C_sp  OutDataType=fixdt(1, 16)  OutScaling=2^0
  Constant5 : Constant  Value=C_ep  OutDataType=fixdt(1, 16)  OutScaling=2^0
  Constant6 : Constant  Value=V_tot  OutDataType=fixdt(1, 16)  OutScaling=2^0
  Constant7 : Constant  Value=C_bv  OutDataType=fixdt(1, 16)  OutScaling=2^0
  Constant8 : Constant  Value=C_hv  OutDataType=fixdt(1, 16)  OutScaling=2^0
  Constant9 : Constant  Value=C_mv  OutDataType=fixdt(1, 16)  OutScaling=2^0
  Demux : Demux  Outputs=16
  Divide : Product  Inputs=*/  OutDataType=fixdt(1, 16)  OutScaling=2^-10
  Product{,1..10} (11 alike) : Product  OutDataType=fixdt(1, 16)  OutScaling=2^0  RndMeth=Zero
  Out1 : Outport  OutDataType=fixdt(1, 16)  OutScaling=2^0
  wires:
  In1/1 -> Demux/1
  Constant1/1 -> Add/1
  Constant2/1 -> Add/2
  Constant3/1 -> Add/3
  Constant4/1 -> Add/4
  Constant5/1 -> Add/5
  Add/1 -> Product2/1
  Demux/1 -> Product2/2
  Demux/2 -> Product/2
  Constant/1 -> Product/1
  Constant7/1 -> Product1/1
  Demux/3 -> Product1/2
  Demux/4 -> Product3/1
  Constant8/1 -> Product3/2
  Constant9/1 -> Product4/1
  Demux/5 -> Product4/2
  Constant10/1 -> Product5/1
  Demux/6 -> Product5/2  "P_ra"
  Constant11/1 -> Product6/2
  Demux/7 -> Product6/1
  Constant13/1 -> Product7/2
  Demux/8 -> Product7/1
  Constant14/1 -> Product8/2
  Demux/9 -> Product8/1
  Constant15/1 -> Product9/2
  Demux/10 -> Product9/1
  Constant16/1 -> Product10/2
  Demux/11 -> Product10/1
  Constant6/1 -> Add1/1
  Product/1 -> Add1/2
  Product2/1 -> Add1/3
  Product1/1 -> Add1/4
  Product3/1 -> Add1/5
  Product4/1 -> Add1/6
  Product5/1 -> Add1/7
  Product6/1 -> Add1/8
  Demux/12 -> Add1/9
  Product7/1 -> Add1/10
  Product8/1 -> Add1/11
  Product9/1 -> Add1/12
  Product10/1 -> Add1/13
  Demux/13 -> Add1/14
  Add1/1 -> Divide/1
  Constant17/1 -> Divide/2
  Constant18/1 -> Add2/1
  Constant19/1 -> Add2/2
  Constant20/1 -> Add2/3
  Constant21/1 -> Add2/4
  Constant22/1 -> Add2/5
  Constant23/1 -> Add2/6
  Constant24/1 -> Add2/7
  Constant25/1 -> Add2/8
  Demux/14 -> Add2/9
  Demux/15 -> Add2/10
  Demux/16 -> Add2/11
  Constant26/1 -> Add2/12
  Constant27/1 -> Add2/13
  Constant28/1 -> Add2/14
  Constant29/1 -> Add2/15
  Constant30/1 -> Add2/16
  Add2/1 -> Add1/15
  Divide/1 -> Out1/1

== system model/A1.13 - P_la ==
  note: P_pv
  note: F_i,l
  In1 : Inport  OutDataType=fixdt(1, 16)  OutScaling=2^0
  Constant : Constant  Value=R_pv  OutDataType=fixdt(1, 16)  OutScaling=2^0
  Constant2 : Constant  Value=C_la  OutDataType=fixdt(1, 16)  OutScaling=2^0
  Demux : Demux  Outputs=2
  Divide : Product  Inputs=*/  OutDataType=fixdt(1, 16)  OutScaling=2^-10
  Divide2 : Product  Inputs=*/  OutDataType=fixdt(1, 16)  OutScaling=2^-10
  Integrator : Integrator  InitialCondition=1
  Subtract : Sum  Inputs=+-  OutDataType=fixdt(1, 16)  OutScaling=2^-10
  Subtract2 : Sum  Inputs=+-  OutDataType=fixdt(1, 16)  OutScaling=2^-10
  Out1 : Outport  OutDataType=fixdt(1, 16)  OutScaling=2^0
  wires:
  In1/1 -> Demux/1
  Demux/1 -> Subtract/1
  Subtract/1 -> Divide/1
  Constant/1 -> Divide/2
  Divide/1 -> Subtract2/1
  Subtract2/1 -> Divide2/1
  Constant2/1 -> Divide2/2
  Divide2/1 -> Integrator/1
  Integrator/1 -> Out1/1, Subtract/2
  Demux/2 -> Subtract2/2

== system model/A1.14 - F_i,l ==
  note: P_la
  note: P_lv
  In1 : Inport  OutDataType=fixdt(1, 16)  OutScaling=2^0
  Constant : Constant  Value=R_la  OutDataType=fixdt(1, 16)  OutScaling=2^0
  Constant1 : Constant  Value=0  OutDataType=fixdt(1, 16)  OutScaling=2^0
  Demux : Demux  Outputs=2
  Divide : Product  Inputs=*/  OutDataType=fixdt(1, 16)  OutScaling=2^-10
  Relational Operator : RelationalOperator  Operator=>  LogicOutDataTypeMode=boolean  LogicDataType=fixdt(0, 8)  OutDataTypeStr=boolean
  Subtract : Sum  Inputs=+-  OutDataType=fixdt(1, 16)  OutScaling=2^-10
  Switch : Switch  Criteria=u2 ~= 0  OutDataType=fixdt(1, 16)  OutScaling=2^0
  Out1 : Outport  OutDataType=fixdt(1, 16)  OutScaling=2^0
  wires:
  In1/1 -> Demux/1
  Demux/1 -> Subtract/1, Relational Operator/1
  Demux/2 -> Subtract/2, Relational Operator/2
  Subtract/1 -> Divide/1
  Constant/1 -> Divide/2
  Divide/1 -> Switch/1
  Constant1/1 -> Switch/3
  Switch/1 -> Out1/1
  Relational Operator/1 -> Switch/2

== system model/A1.15 - V_lv ==
  note: F_i,l
  note: F_o,l
  In1 : Inport  OutDataType=fixdt(1, 16)  OutScaling=2^0
  Demux : Demux  Outputs=2
  Integrator : Integrator  InitialCondition=1
  Subtract : Sum  Inputs=+-  OutDataType=fixdt(1, 16)  OutScaling=2^-10
  Out1 : Outport  OutDataType=fixdt(1, 16)  OutScaling=2^0
  wires:
  In1/1 -> Demux/1
  Demux/1 -> Subtract/1
  Demux/2 -> Subtract/2
  Subtract/1 -> Integrator/1
  Integrator/1 -> Out1/1

== system model/A1.16 - F_o,l ==
  note: P_max_lv
  note: P_sa
  note: R_lv
  In1 : Inport  OutDataType=fixdt(1, 16)  OutScaling=2^0
  Constant : Constant  Value=0  OutDataType=fixdt(1, 16)  OutScaling=2^0
  Demux : Demux  Outputs=3
  Divide : Product  Inputs=*/  OutDataType=fixdt(1, 16)  OutScaling=2^-10
  Relational Operator : RelationalOperator  Operator=>  LogicOutDataTypeMode=boolean  LogicDataType=fixdt(0, 8)  OutDataTypeStr=boolean
  Subtract : Sum  Inputs=+-  OutDataType=fixdt(1, 16)  OutScaling=2^-10
  Switch : Switch  OutDataType=fixdt(1, 16)  OutScaling=2^0
  Out1 : Outport  OutDataType=fixdt(1, 16)  OutScaling=2^0
  wires:
  In1/1 -> Demux/1
  Demux/1 -> Subtract/1, Relational Operator/1
  Demux/2 -> Subtract/2, Relational Operator/2
  Subtract/1 -> Divide/1
  Demux/3 -> Divide/2
  Switch/1 -> Out1/1
  Divide/1 -> Switch/1
  Constant/1 -> Switch/3
  Relational Operator/1 -> Switch/2

== system model/A1.17 - R_lv ==
  note: P_max_lv
  In1 : Inport  OutDataType=fixdt(1, 16)  OutScaling=2^0
  Constant : Constant  Value=k_r_lv  OutDataType=fixdt(1, 16)  OutScaling=2^0
  Product : Product  OutDataType=fixdt(1, 16)  OutScaling=2^0  RndMeth=Zero
  Out1 : Outport  OutDataType=fixdt(1, 16)  OutScaling=2^0
  wires:
  In1/1 -> Product/1
  Constant/1 -> Product/2
  Product/1 -> Out1/1

== system model/A1.18 - P_max_lv ==
  note: fi
  note: V_lv
  In1 : Inport  OutDataType=fixdt(1, 16)  OutScaling=2^0
  Constant1 : Constant  Value=V_u_lv  OutDataType=fixdt(1, 16)  OutScaling=2^0
  Constant2 : Constant  OutDataType=fixdt(1, 16)  OutScaling=2^0
  Constant3 : Constant  Value=k_e_lv  OutDataType=fixdt(1, 16)  OutScaling=2^0
  Constant4 : Constant  Value=P_o_lv  OutDataType=fixdt(1, 16)  OutScaling=2^0
  Demux : Demux  Outputs=3
  Math Function : Math  OutDataType=fixdt(1, 16)  OutScaling=2^0  SaturateOnIntegerOverflow=on
  Product : Product  Inputs=6  OutDataType=fixdt(1, 16)  OutScaling=2^0  RndMeth=Zero
  Product1 : Product  OutDataType=fixdt(1, 16)  OutScaling=2^0  RndMeth=Zero
  Subtract : Sum  Inputs=+-  OutDataType=fixdt(1, 16)  OutScaling=2^-10
  Subtract1 : Sum  Inputs=+-  OutDataType=fixdt(1, 16)  OutScaling=2^-10
  Subtract2 : Sum  Inputs=+-  OutDataType=fixdt(1, 16)  OutScaling=2^-10
  Out1 : Outport  OutDataType=fixdt(1, 16)  OutScaling=2^0
  wires:
  In1/1 -> Demux/1
  Demux/1 -> Product/1, Subtract1/2
  Demux/2 -> Subtract/1, Product1/2
  Constant1/1 -> Subtract/2
  Subtract/1 -> Product/3
  Constant2/1 -> Subtract1/1, Subtract2/2
  Subtract1/1 -> Product/4
  Constant3/1 -> Product1/1
  Product1/1 -> Math Function/1
  Math Function/1 -> Subtract2/1
  Subtract2/1 -> Product/6
  Product/1 -> Out1/1
  Constant4/1 -> Product/5
  Demux/3 -> Product/2

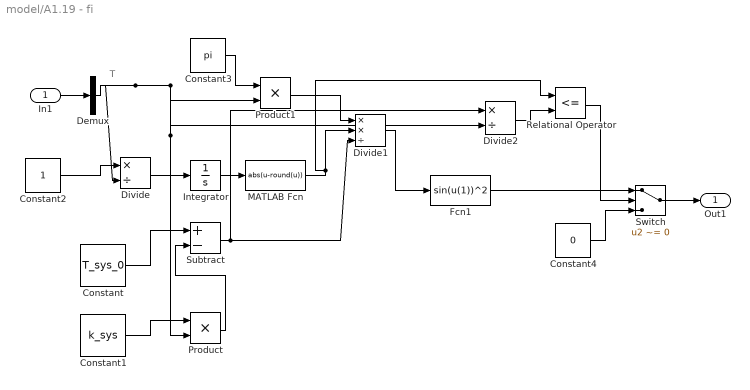
== system model/A1.19 - fi ==
  note: T
  In1 : Inport  OutDataType=fixdt(1, 16)  OutScaling=2^0
  Constant : Constant  Value=T_sys_0  OutDataType=fixdt(1, 16)  OutScaling=2^0
  Constant1 : Constant  Value=k_sys  OutDataType=fixdt(1, 16)  OutScaling=2^0
  Constant2 : Constant  OutDataType=fixdt(1, 16)  OutScaling=2^0
  Constant3 : Constant  Value=pi  OutDataType=fixdt(1, 16)  OutScaling=2^0
  Constant4 : Constant  Value=0  OutDataType=fixdt(1, 16)  OutScaling=2^0
  Demux : Demux  Outputs=1
  Divide : Product  Inputs=*/  OutDataType=fixdt(1, 16)  OutScaling=2^-10
  Divide1 : Product  Inputs=**/  OutDataType=fixdt(1, 16)  OutScaling=2^-10
  Divide2 : Product  Inputs=*/  OutDataType=fixdt(1, 16)  OutScaling=2^-10
  Fcn1 : Fcn  Expr=sin(u(1))^2
  Integrator : Integrator  InitialCondition=1
  MATLAB Fcn : MATLABFcn  MATLABFcn=abs(u-round(u))
  Product : Product  OutDataType=fixdt(1, 16)  OutScaling=2^0  RndMeth=Zero
  Product1 : Product  OutDataType=fixdt(1, 16)  OutScaling=2^0  RndMeth=Zero
  Relational Operator : RelationalOperator  Operator=<=  LogicOutDataTypeMode=boolean  LogicDataType=fixdt(0, 8)  OutDataTypeStr=boolean
  Subtract : Sum  Inputs=+-  OutDataType=fixdt(1, 16)  OutScaling=2^-10
  Switch : Switch  Criteria=u2 ~= 0  OutDataType=fixdt(1, 16)  OutScaling=2^0
  Out1 : Outport  OutDataType=fixdt(1, 16)  OutScaling=2^0
  wires:
  Constant/1 -> Subtract/1
  Constant1/1 -> Product/1
  In1/1 -> Demux/1
  Demux/1 -> Divide/2, Product1/2, Product/2, Divide2/2
  Product/1 -> Subtract/2
  Constant2/1 -> Divide/1
  Divide/1 -> Integrator/1
  Constant3/1 -> Product1/1
  Product1/1 -> Divide1/1
  MATLAB Fcn/1 -> Divide1/2, Relational Operator/1
  Subtract/1 -> Divide1/3, Divide2/1
  Divide1/1 -> Fcn1/1
  Divide2/1 -> Relational Operator/2
  Relational Operator/1 -> Switch/2
  Fcn1/1 -> Switch/1
  Constant4/1 -> Switch/3
  Switch/1 -> Out1/1
  Integrator/1 -> MATLAB Fcn/1

== system model/A1.2 - F_pa ==
  note: P pa
  note: P pp
  In1 : Inport  OutDataType=fixdt(1, 16)  OutScaling=2^0
  Constant : Constant  Value=R_pa  OutDataType=fixdt(1, 16)  OutScaling=2^0
  Constant1 : Constant  Value=L_pa  OutDataType=fixdt(1, 16)  OutScaling=2^0
  Demux : Demux  Outputs=2
  Divide : Product  Inputs=*/  OutDataType=fixdt(1, 16)  OutScaling=2^-10
  Integrator : Integrator  InitialCondition=1
  Product : Product  OutDataType=fixdt(1, 16)  OutScaling=2^0  RndMeth=Zero
  Subtract : Sum  Inputs=+--  OutDataType=fixdt(1, 16)  OutScaling=2^-10
  Out1 : Outport  OutDataType=fixdt(1, 16)  OutScaling=2^0
  wires:
  In1/1 -> Demux/1
  Demux/1 -> Subtract/1
  Demux/2 -> Subtract/2
  Constant/1 -> Product/2
  Product/1 -> Subtract/3
  Subtract/1 -> Divide/1
  Divide/1 -> Integrator/1
  Integrator/1 -> Out1/1, Product/1
  Constant1/1 -> Divide/2

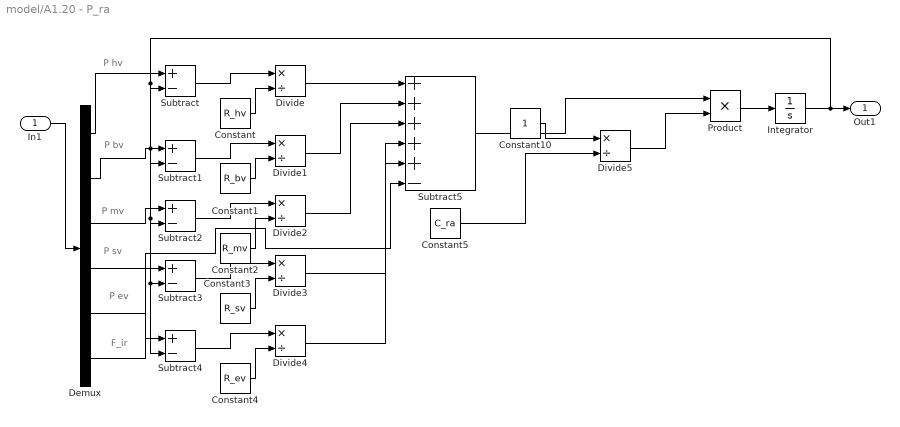
== system model/A1.20 - P_ra ==
  note: P hv
  note: P bv
  note: P mv
  note: P sv
  note: P ev
  note: F_ir
  In1 : Inport  OutDataType=fixdt(1, 16)  OutScaling=2^0
  Constant : Constant  Value=R_hv  OutDataType=fixdt(1, 16)  OutScaling=2^0
  Constant1 : Constant  Value=R_bv  OutDataType=fixdt(1, 16)  OutScaling=2^0
  Constant10 : Constant  OutDataType=fixdt(1, 16)  OutScaling=2^0
  Constant2 : Constant  Value=R_mv  OutDataType=fixdt(1, 16)  OutScaling=2^0
  Constant3 : Constant  Value=R_sv  OutDataType=fixdt(1, 16)  OutScaling=2^0
  Constant4 : Constant  Value=R_ev  OutDataType=fixdt(1, 16)  OutScaling=2^0
  Constant5 : Constant  Value=C_ra  OutDataType=fixdt(1, 16)  OutScaling=2^0
  Demux : Demux  Outputs=6
  Divide{,1..5} (6 alike) : Product  Inputs=*/  OutDataType=fixdt(1, 16)  OutScaling=2^-10
  Integrator : Integrator  InitialCondition=1
  Product : Product  OutDataType=fixdt(1, 16)  OutScaling=2^0  RndMeth=Zero
  Subtract{,1..4} (5 alike) : Sum  Inputs=+-  OutDataType=fixdt(1, 16)  OutScaling=2^-10
  Subtract5 : Sum  Inputs=+++++-  OutDataType=fixdt(1, 16)  OutScaling=2^-10
  Out1 : Outport  OutDataType=fixdt(1, 16)  OutScaling=2^0
  wires:
  In1/1 -> Demux/1
  Constant/1 -> Divide/2
  Subtract/1 -> Divide/1
  Constant1/1 -> Divide1/2
  Subtract1/1 -> Divide1/1
  Subtract2/1 -> Divide2/1
  Subtract3/1 -> Divide3/1
  Subtract4/1 -> Divide4/1
  Constant10/1 -> Divide5/1
  Subtract5/1 -> Product/1
  Divide5/1 -> Product/2
  Product/1 -> Integrator/1
  Integrator/1 -> Out1/1, Subtract/2, Subtract1/2, Subtract2/2, Subtract3/2, Subtract4/2
  Constant5/1 -> Divide5/2
  Demux/1 -> Subtract/1
  Demux/2 -> Subtract1/1
  Demux/3 -> Subtract2/1
  Demux/4 -> Subtract3/1
  Demux/5 -> Subtract4/1
  Constant2/1 -> Divide2/2
  Constant3/1 -> Divide3/2
  Constant4/1 -> Divide4/2
  Demux/6 -> Subtract5/6
  Divide4/1 -> Subtract5/5
  Divide3/1 -> Subtract5/4
  Divide2/1 -> Subtract5/3
  Divide1/1 -> Subtract5/2
  Divide/1 -> Subtract5/1

== system model/A1.21 - F_i,r ==
  note: P_ra
  note: P_rv
  In1 : Inport  OutDataType=fixdt(1, 16)  OutScaling=2^0
  Constant : Constant  Value=0  OutDataType=fixdt(1, 16)  OutScaling=2^0
  Constant1 : Constant  Value=R_ra  OutDataType=fixdt(1, 16)  OutScaling=2^0
  Demux : Demux  Outputs=2
  Divide : Product  Inputs=*/  OutDataType=fixdt(1, 16)  OutScaling=2^-10
  Relational Operator : RelationalOperator  Operator=>  LogicOutDataTypeMode=boolean  LogicDataType=fixdt(0, 8)  OutDataTypeStr=boolean
  Subtract : Sum  Inputs=+-  OutDataType=fixdt(1, 16)  OutScaling=2^-10
  Switch : Switch  OutDataType=fixdt(1, 16)  OutScaling=2^0
  Out1 : Outport  OutDataType=fixdt(1, 16)  OutScaling=2^0
  wires:
  In1/1 -> Demux/1
  Demux/1 -> Subtract/1, Relational Operator/1
  Demux/2 -> Subtract/2, Relational Operator/2
  Subtract/1 -> Divide/1
  Switch/1 -> Out1/1
  Divide/1 -> Switch/1
  Constant/1 -> Switch/3
  Relational Operator/1 -> Switch/2
  Constant1/1 -> Divide/2

== system model/A1.22 - V_r,v ==
  note: F_i,r
  note: F_o,r
  In1 : Inport  OutDataType=fixdt(1, 16)  OutScaling=2^0
  Demux : Demux  Outputs=2
  Integrator : Integrator  InitialCondition=1
  Subtract : Sum  Inputs=+-  OutDataType=fixdt(1, 16)  OutScaling=2^-10
  Out1 : Outport  OutDataType=fixdt(1, 16)  OutScaling=2^0
  wires:
  In1/1 -> Demux/1
  Demux/1 -> Subtract/1
  Demux/2 -> Subtract/2
  Subtract/1 -> Integrator/1
  Integrator/1 -> Out1/1

== system model/A1.23- F_o,r ==
  note: P_max_rv
  note: P_pa
  note: R_rv
  In1 : Inport  OutDataType=fixdt(1, 16)  OutScaling=2^0
  Constant : Constant  Value=0  OutDataType=fixdt(1, 16)  OutScaling=2^0
  Demux : Demux  Outputs=3
  Divide : Product  Inputs=*/  OutDataType=fixdt(1, 16)  OutScaling=2^-10
  Relational Operator : RelationalOperator  Operator=>  LogicOutDataTypeMode=boolean  LogicDataType=fixdt(0, 8)  OutDataTypeStr=boolean
  Subtract : Sum  Inputs=+-  OutDataType=fixdt(1, 16)  OutScaling=2^-10
  Switch : Switch  OutDataType=fixdt(1, 16)  OutScaling=2^0
  Out1 : Outport  OutDataType=fixdt(1, 16)  OutScaling=2^0
  wires:
  In1/1 -> Demux/1
  Demux/1 -> Subtract/1, Relational Operator/1
  Demux/2 -> Subtract/2, Relational Operator/2
  Subtract/1 -> Divide/1
  Demux/3 -> Divide/2
  Switch/1 -> Out1/1
  Divide/1 -> Switch/1
  Constant/1 -> Switch/3
  Relational Operator/1 -> Switch/2

== system model/A1.24 - R_r,v ==
  note: P_max_rv
  In1 : Inport  OutDataType=fixdt(1, 16)  OutScaling=2^0
  Constant : Constant  Value=k_r_rv  OutDataType=fixdt(1, 16)  OutScaling=2^0
  Product : Product  OutDataType=fixdt(1, 16)  OutScaling=2^0  RndMeth=Zero
  Out1 : Outport  OutDataType=fixdt(1, 16)  OutScaling=2^0
  wires:
  In1/1 -> Product/1
  Constant/1 -> Product/2
  Product/1 -> Out1/1

== system model/A1.25 - P_max_rv ==
  note: fi
  note: V_rv
  In1 : Inport  OutDataType=fixdt(1, 16)  OutScaling=2^0
  Constant1 : Constant  Value=V_u_rv  OutDataType=fixdt(1, 16)  OutScaling=2^0
  Constant2 : Constant  OutDataType=fixdt(1, 16)  OutScaling=2^0
  Constant3 : Constant  Value=k_e_rv  OutDataType=fixdt(1, 16)  OutScaling=2^0
  Constant4 : Constant  Value=P_o_rv  OutDataType=fixdt(1, 16)  OutScaling=2^0
  Demux : Demux  Outputs=3
  Math Function : Math  OutDataType=fixdt(1, 16)  OutScaling=2^0  SaturateOnIntegerOverflow=on
  Product : Product  Inputs=6  OutDataType=fixdt(1, 16)  OutScaling=2^0  RndMeth=Zero
  Product1 : Product  OutDataType=fixdt(1, 16)  OutScaling=2^0  RndMeth=Zero
  Subtract : Sum  Inputs=+-  OutDataType=fixdt(1, 16)  OutScaling=2^-10
  Subtract1 : Sum  Inputs=+-  OutDataType=fixdt(1, 16)  OutScaling=2^-10
  Subtract2 : Sum  Inputs=+-  OutDataType=fixdt(1, 16)  OutScaling=2^-10
  Out1 : Outport  OutDataType=fixdt(1, 16)  OutScaling=2^0
  wires:
  In1/1 -> Demux/1
  Demux/1 -> Product/1, Subtract1/2
  Demux/2 -> Subtract/1, Product1/2
  Constant1/1 -> Subtract/2
  Subtract/1 -> Product/3
  Constant2/1 -> Subtract1/1, Subtract2/2
  Subtract1/1 -> Product/4
  Constant3/1 -> Product1/1
  Product1/1 -> Math Function/1
  Math Function/1 -> Subtract2/1
  Subtract2/1 -> Product/6
  Product/1 -> Out1/1
  Constant4/1 -> Product/5
  Demux/3 -> Product/2
